simulink model "td3"  (R2014a)
settings: Solver=ode45  StartTime=0.0  StopTime=10.0  RelTol=1e-3
libraries: simulink x1
settings Model: Creator=elkhadiy  LastModifiedBy=elkhadiy

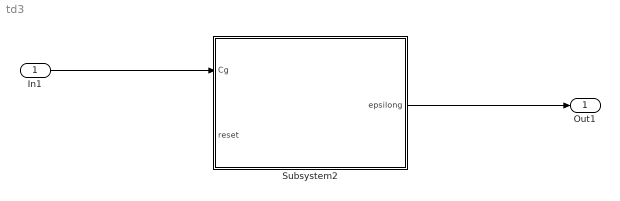
== system td3 ==
  In1 : Inport
  Subsystem2 : Subsystem
  Out1 : Outport
  wires:
  In1/1 -> Subsystem2/1(Cg)
  Subsystem2/1(epsilong) -> Out1/1

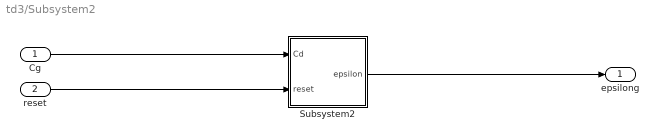
== system td3/Subsystem2 ==
  Cg : Inport
  reset : Inport  Port=2
  Subsystem2 : Subsystem
  epsilong : Outport
  wires:
  Cg/1 -> Subsystem2/1(Cd)
  Subsystem2/1(epsilon) -> epsilong/1
  reset/1 -> Subsystem2/2(reset)

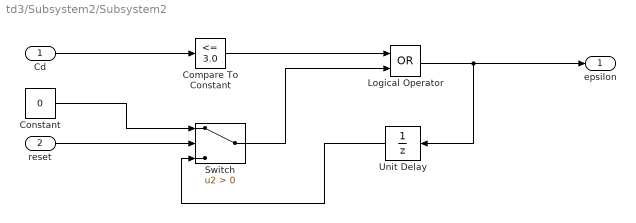
== system td3/Subsystem2/Subsystem2 ==
  Cd : Inport
  reset : Inport  Port=2
  Compare To Constant : simulink/Logic and Bit Operations/Compare To Constant  relop=<=  const=3.0  OutDataTypeStr=boolean
  Constant : Constant  Value=0
  Logical Operator : Logic  Operator=OR  AllPortsSameDT=off  OutDataTypeStr=boolean
  Switch : Switch  Criteria=u2 > Threshold
  Unit Delay : UnitDelay  SampleTime=-1
  epsilon : Outport
  wires:
  Unit Delay/1 -> Switch/3
  Compare To Constant/1 -> Logical Operator/1
  Cd/1 -> Compare To Constant/1
  Logical Operator/1 -> epsilon/1, Unit Delay/1
  Switch/1 -> Logical Operator/2
  reset/1 -> Switch/2
  Constant/1 -> Switch/1
